simulink model "controlled_PID_from_ISO"  (Simulink 7.9)
settings: Solver=ode45  StartTime=0  StopTime=4  FixedStep=0.001  MinStep=0.0001  RelTol=1e-3
values from neighbouring files (symbols this model uses):
  alpha = 5.59E-4    (= 0.000559)    [IS_o.m]
  beta_r = 16.77E-4    (= 0.001677)    [IS_o.m]
  beta_rr = 0    [IS_o.m]
  force_torque_limit_bottom = -1* force_torque_limit_top    (= -28.4)    [IS_o.m]
  force_torque_limit_top = 28.4    [IS_o.m]
undefined symbols (not defined in the file or in its folder): controller_step_onoff, dfilt, disturb_ampl, fdesignblkfcn, gcbh, k_d, k_i, k_p, step_time
libraries: dsparch4 x1
settings Model: Creator=compiaffe  LastModifiedBy=compiaffe

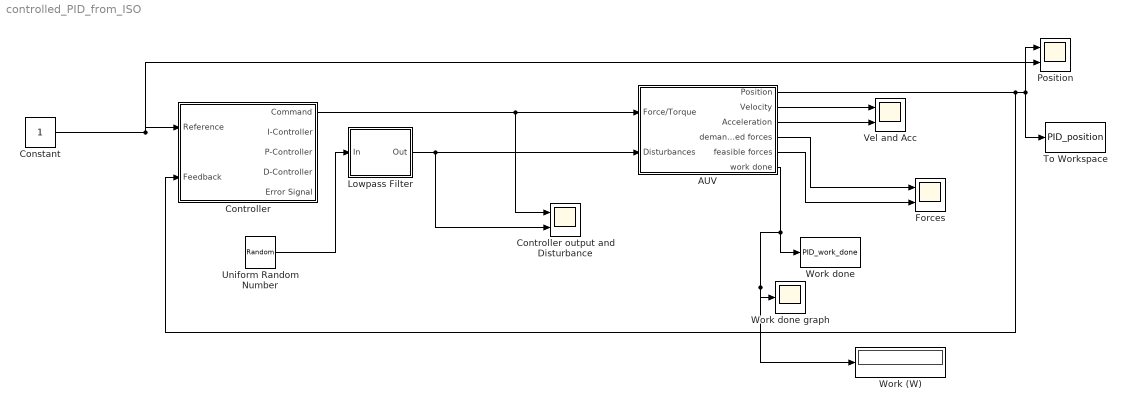
== system controlled_PID_from_ISO ==
  AUV : Subsystem
  Constant : Constant
  Controller : Subsystem
  Controller output and Disturbance : Scope  NumInputPorts=2
      settings: TickLabels=on  ShowLegends=on  YMin=-5e+12~-0.105  YMax=8.5e+13~-0.095  SaveName=ScopeData4  MaxDataPoints=500000  SampleTime=1
  Forces : Scope  NumInputPorts=2
      settings: TickLabels=on  ShowLegends=on  YMin=-0.00325~-0.00325  YMax=0.00125~0.00125  SaveName=ScopeData3  MaxDataPoints=500000  SampleTime=1
  Lowpass Filter : Subsystem  DialogController=fdesignblkfcn  DialogControllerArgs=DataTag1  InitFcn=fdesignblkfcn(gcbh, {'InitFcn'});
      settings: CopyFcn=fdesignblkfcn(gcbh, {'CopyFcn'});
      mask Type: Lowpass Filter
      mask Description: Design a lowpass filter
      mask Help: helpview(mapfilelocation('dsp'), 'dsplowpassfilter');
      mask Display: disp('Lowpass')
  Position : Scope  NumInputPorts=2
      settings: TickLabels=on  ShowLegends=on  TimeRange=10  YMin=0.95~0.95  YMax=1.05~1.05  MaxDataPoints=500000  SampleTime=1
  To Workspace : ToWorkspace  VariableName=PID_position  SampleTime=-1  SaveFormat=Timeseries
  Uniform Random Number : UniformRandomNumber  Minimum=-1*disturb_ampl  Maximum=disturb_ampl  SampleTime=0.1
  Vel and Acc : Scope  NumInputPorts=2
      settings: TickLabels=on  ShowLegends=on  YMin=-100~-5e+12  YMax=90~8.5e+13  SaveName=ScopeData6  MaxDataPoints=500000  SampleTime=1
  Work (W) : Display
  Work done : ToWorkspace  VariableName=PID_work_done  SampleTime=-1  SaveFormat=Timeseries
      settings: MaxDataPoints=1
  Work done graph : Scope
      settings: TimeRange=0.16  SaveName=ScopeData5
  wires:
  AUV/1(Position) -> Position/1, To Workspace/1, Controller/2(Feedback)
  AUV/2(Velocity) -> Vel and Acc/1
  AUV/3(Acceleration) -> Vel and Acc/2
  AUV/4(demanded forces) -> Forces/1
  AUV/5(feasible forces) -> Forces/2
  Controller/1(Command) -> AUV/1(Force/Torque), Controller output and Disturbance/1
  Constant/1 -> Controller/1(Reference), Position/2
  Lowpass Filter/1(Out) -> AUV/2(Disturbances), Controller output and Disturbance/2
  AUV/6(work done) -> Work done/1, Work done graph/1, Work (W)/1
  Uniform Random Number/1 -> Lowpass Filter/1(In)

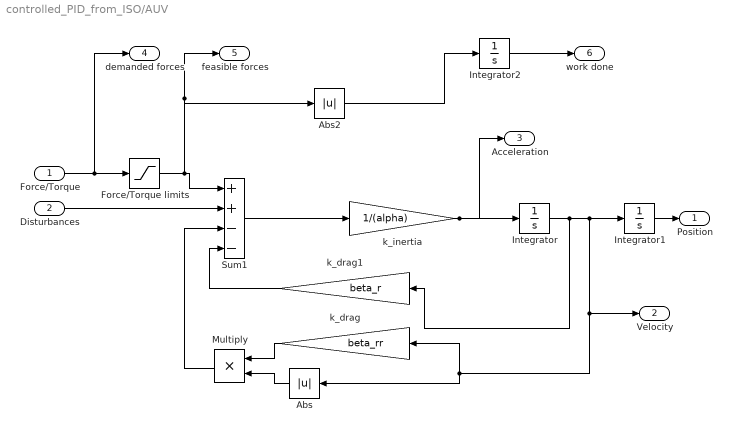
== system controlled_PID_from_ISO/AUV ==
  Force/Torque : Inport
  Disturbances : Inport  Port=2
  Abs : Abs
  Abs2 : Abs
  Force/Torque limits : Saturate  UpperLimit=force_torque_limit_top  LowerLimit=force_torque_limit_bottom
  Integrator : Integrator
  Integrator1 : Integrator
  Integrator2 : Integrator
  Multiply : Product  Inputs=**
  Sum1 : Sum  Inputs=++--
  k_drag : Gain  Gain=beta_rr
  k_drag1 : Gain  Gain=beta_r
  k_inertia : Gain  Gain=1/(alpha)
  Position : Outport
  Velocity : Outport  Port=2
  Acceleration : Outport  Port=3
  demanded forces : Outport  Port=4
  feasible forces : Outport  Port=5
  work done : Outport  Port=6
  wires:
  k_drag1/1 -> Sum1/4
  Abs/1 -> Multiply/2
  k_inertia/1 -> Integrator/1, Acceleration/1
  Sum1/1 -> k_inertia/1
  Multiply/1 -> Sum1/3
  k_drag/1 -> Multiply/1
  Integrator1/1 -> Position/1
  Integrator/1 -> Integrator1/1, Velocity/1, k_drag/1, Abs/1, k_drag1/1
  Integrator2/1 -> work done/1
  Disturbances/1 -> Sum1/2
  Force/Torque/1 -> Force/Torque limits/1, demanded forces/1
  Force/Torque limits/1 -> Sum1/1, feasible forces/1, Abs2/1
  Abs2/1 -> Integrator2/1

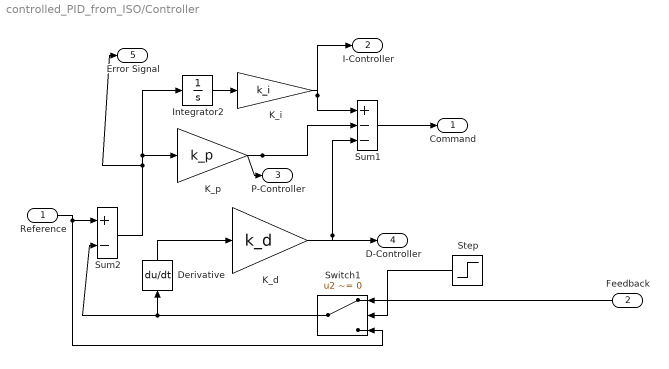
== system controlled_PID_from_ISO/Controller ==
  Reference : Inport
  Feedback : Inport  Port=2
  Derivative : Derivative
  Integrator2 : Integrator
  K_d : Gain  Gain=k_d
  K_i : Gain  Gain=k_i
  K_p : Gain  Gain=k_p
  Step : Step  Time=step_time  After=controller_step_onoff  SampleTime=0
  Sum1 : Sum  Inputs=+--
  Sum2 : Sum  Inputs=+-
  Switch1 : Switch  Criteria=u2 ~= 0  Threshold=0.5
  Command : Outport
  I-Controller : Outport  Port=2
  P-Controller : Outport  Port=3
  D-Controller : Outport  Port=4
  Error Signal : Outport  Port=5
  wires:
  Integrator2/1 -> K_i/1
  K_i/1 -> Sum1/1, I-Controller/1
  K_d/1 -> D-Controller/1, Sum1/3
  Derivative/1 -> K_d/1
  K_p/1 -> Sum1/2, P-Controller/1
  Switch1/1 -> Derivative/1, Sum2/2
  Step/1 -> Switch1/2
  Sum1/1 -> Command/1
  Feedback/1 -> Switch1/1
  Reference/1 -> Sum2/1, Switch1/3
  Sum2/1 -> Integrator2/1, K_p/1, Error Signal/1

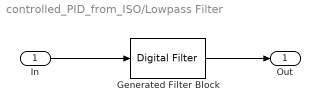
== system controlled_PID_from_ISO/Lowpass Filter ==
  In : Inport
  Generated Filter Block : dsparch4/Digital Filter  Tag=BlockMethodSubSystem  TypePopup=FIR (all zeros)  IIRFiltStruct=Direct form II transposed  AllPoleFiltStruct=Direct form  FIRFiltStruct=Direct form  CoeffSource=Specify via dialog  NumCoeffs=[0.000431228805668185 -0.000136602287088064 -0.00016280775386646 -0.000213241909853283 -0.000284687363806192 -0.000374516009099117 -0.000480818418670433 -0.000601393619555318 -0.000734165931484247 -0.000876403883770064 -0.00102533176118301 -0.0011774202324644 -0.00132911388476705 -0.00147620005958787 -0.00161460858802971 -0.00173980006364118 -0.0018476525118686 -0.00193383744375592 -0.00199475266914396 -0.00202686625134454 -0.00202770407616183 -0.00199510576379253 -0.00192823618575947 -0.00182672421853782 -0.00169173944385792 -0.00152495466694567 -0.00132967859811586 -0.00110960374752446 -0.000870069535307166 -0.000616439126781768 -0.000355642278733587 -9.4025237041963e-05 0.000160499194491233 0.000401835791686176 0.000621586009553478 0.000814422287655452 0.000975143247415437 0.00109642639378899 0.00117618193456041 0.00121138001473177 0.00120130238819034 0.00114585859936874 0.00104725011274568 0.000908630676759415 0.000735087615949306 0.0005325893551465 0.00030856974248692 7.10316410966622e-05 -0.000171126128377671 -0.000408942053911337 -0.000633243940616709 -0.000835394578578259 -0.00100725532294377 -0.00114183196418552 -0.00123325943615467 -0.00127731356409512 -0.0012713822317219 -0.00121481980820665 -0.00110882559919418 -0.000956593592831169 -0.000763116621661031 -0.000535148191727726 -0.000280881367634712 -9.74379693077524e-06 0.000267949210637483 0.000541406682321087 0.000799687035391103 0.00103228098528323 0.00122909694439026 0.00138193583768818 0.00148296047454369 0.00152730300268713 0.00151187862307046 0.00143543403108213 0.00129948209904952 0.00110787795733382 0.000866860762125757 0.000584651340612045 0.000271424152475853 -6.12267715454403e-05 -0.000400522469569281 -0.000733137167577309 -0.00104557133252268 -0.0013248224411933 -0.00155877510970958 -0.0017368396855896 -0.00185029175232458 -0.00189278941222409 -0.00186058188210732 -0.00175284946353553 -0.00157170555182596 -0.00132229868247862 -0.00101258628808832 -0.000653229951473376 -0.000257133893125731 0.000160900946134091 0.000584824488230154 0.000997785832298983 0.0013829638880681 0.00172406235236673 0.00200615053187214 0.00221607387458729 0.00234335365278959 0.00238032084715768 0.00232267496653283 0.00217008456917843 0.00192544015477923 0.00159586235398644 0.0011919773856774 0.000727684648565952 0.000219628087709647 -0.000313151503174279 -0.000850081302091175 -0.00136972196333766 -0.00185070924646425 -0.00227250258461024 -0.0026163190737268 -0.00286583812524897 -0.00300802334955098 -0.00303366613945877 -0.00293795189867248 -0.00272071923919297 -0.00238668863177909 -0.00194536225835817 -0.00141087205368172 -0.000801513847225379 -0.000139226672040647 0.000551225601044681 0.00124310164106882 0.0019087112506164 0.0025204161586262 0.00305179843106707 0.00347871695997063 0.00378032622280255 0.00394003419678519 0.00394631667287531 0.00379336586355881 0.00348138703260602 0.00301713027929543 0.00241343767984306 0.00168924628719879 0.000869125470106732 -1.78382305600351e-05 -0.000938669614218368 -0.00185776966003825 -0.00273817162576229 -0.00354308291222116 -0.00423715992729646 -0.0047880640402349 -0.00516772823296829 -0.00535374516889495 -0.00533035928692585 -0.00508946666331473 -0.00463112535481425 -0.00396400914222732 -0.00310532699692373 -0.00208063906069913 -0.000923126294590344 0.000327237438330571 0.0016250302977901 0.00292076330845146 0.00416269211995028 0.0052985454011026 0.00627759198964577 0.0070525404853697 0.00758160563858557 0.00783017258112652 0.00777259762831246 0.00739351856588311 0.00668903399819691 0.00566729454789476 0.00434908072651734 0.00276752104253661 0.000967647306999036 -0.000994395624212899 -0.00305293211730403 -0.00513434269204745 -0.00715906459760176 -0.0090440813754647 -0.0107053900973804 -0.0120606562207325 -0.0130318871269346 -0.0135481921569369 -0.0135482432278406 -0.012982643845528 -0.0118158668726417 -0.0100279591465396 -0.00761567625520311 -0.0045932767955694 -0.000992646200604788 0.00313696613136924 0.0077298954282795 ...(+4491 chars)]  DenCoeffs=[1 0.1]  BiQuadCoeffs=[1 0.3 0.4 1 0.1 0.2]  LatticeCoeffs=[0.2 0.4]  denIgnore=on  FiltPerSampPopup=One filter per frame  IC=0  ICnum=0  ICden=0  roundingMode=Floor  overflowMode=off  ScaleValues=1  scaleValueFracLength=14  stageInFracLength=15  stageOutFracLength=15  FilterSource=Specify via dialog  dfiltObjectName=dfilt.dffir([1 2 1])  InputProcessing=Columns as channels (frame based)
  Out : Outport
  wires:
  In/1 -> Generated Filter Block/1
  Generated Filter Block/1 -> Out/1
